simulink model "raspberrypi_robotaurus3"  (R2014a)
settings: Solver=FixedStepDiscrete  StartTime=0.0  StopTime=inf  RelTol=1e-3
undefined symbols (not defined in the file or in its folder): Rec, SDTV
libraries: embdlinuxlib x4, visionconversions x1
PreSaveFcn:
  | set_param(gcs, 'Location',[35 56 895 605])
settings Model: SimulationMode=external  ExtModeTrigDuration=100  Creator=The MathWorks Inc.  LastModifiedBy=Alejandro
settings DataIOCC: SignalLoggingSaveFormat=ModelDataLogs
settings OptimizationCC: ExpressionDepthLimit=2147483647  OptimizeModelRefInitCode=on  LifeSpan=Inf
settings DebuggingCC: UnderspecifiedInitializationDetection=Classic  SolverPrmCheckMsg=none  FcnCallInpInsideContextMsg=EnableAllAsWarning  StateNameClashWarn=warning
settings HardwareCC: ProdLargestAtomicInteger=Long  ProdLargestAtomicFloat=Double  ProdEndianess=LittleEndian  ProdHWDeviceType=ARM Compatible->ARM Cortex
settings RTWCC: SystemTargetFile=realtime.tlc  GenerateMakefile=off  TemplateMakefile=realtime.tmf  Description=Run on Target Hardware  RTWVerbose=off  ProcessScript=realtime_make_rtw_hook
settings CodeAppCC: CustomSymbolStrType=$N$R$M  InternalIdentifier=Classic
settings STFCustomTargetCC: TargetLibSuffix=.a  GenerateSampleERTMain=on  ConcurrentExecutionCompliant=off  GeneratePreprocessorConditionals=Use local settings  ERTCustomFileBanners=on  SupportNonInlinedSFcns=off  SupportVariableSizeSignals=on  MATLABClassNameForMDSCustomization=Simulink.SoftwareTarget.ERTCustomization  GRTInterface=off  SystemTargetFile=realtime.tlc
settings ERTTargetCC: CombineOutputUpdateFcns=off  SupportContinuousTime=on  SupportVariableSizeSignals=on  ExtMode=on  ExtModeMexArgs='169.254.0.2' 0 17725 5  ERTSrcFileBannerTemplate=realtime_code_template.cgt  ERTHdrFileBannerTemplate=realtime_code_template.cgt  ERTDataSrcFileTemplate=realtime_code_template.cgt  ERTDataHdrFileTemplate=realtime_code_template.cgt  ERTCustomFileTemplate=realtime_file_process.tlc

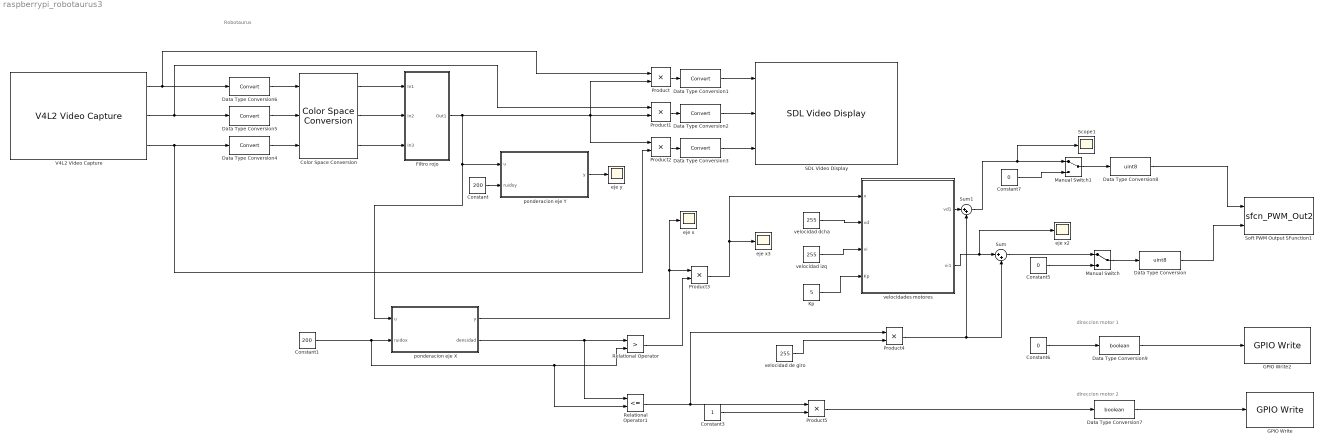
== system raspberrypi_robotaurus3 ==
  note: direccion motor 1
  note: direccion motor 2
  note: Robotaurus
  Color Space Conversion : visionconversions/Color Space  Conversion  conversion=Obsolete  conversionActive=R'G'B' to HSV  wp_str=D65  rec=Rec. 601 (SDTV)  sys=1125/60/2:1  imagePorts=Separate color signals
  Constant : Constant  Value=200
  Constant1 : Constant  Value=200
  Constant3 : Constant
  Constant5 : Constant  Value=0
  Constant6 : Constant  Value=0
  Constant7 : Constant  Value=0
  Data Type Conversion : DataTypeConversion  OutDataTypeStr=uint8
  Data Type Conversion{1..6} (6 alike) : DataTypeConversion
  Data Type Conversion7 : DataTypeConversion  OutDataTypeStr=boolean
  Data Type Conversion8 : DataTypeConversion  OutDataTypeStr=uint8
  Data Type Conversion9 : DataTypeConversion  OutDataTypeStr=boolean
  Filtro rojo : Subsystem
  GPIO Write : embdlinuxlib/GPIO Write  board=Model B Rev2  gpio=4  direction=Output  blockPlatform=Raspberry Pi
  GPIO Write2 : embdlinuxlib/GPIO Write  board=Model B Rev2  gpio=25  direction=Output  blockPlatform=Raspberry Pi
  Kp : Constant  Value=5
  Manual Switch : ManualSwitch
  Manual Switch1 : ManualSwitch
  Product{,1..5} (6 alike) : Product
  Relational Operator : RelationalOperator  Operator=>  OutDataTypeStr=boolean
  Relational Operator1 : RelationalOperator  Operator=<=  OutDataTypeStr=boolean
  SDL Video Display : embdlinuxlib/SDL Video Display  pixelFormat=RGB  pixelOrder=Planar  rowMajor=on  blockPlatform=Raspberry Pi
  Scope1 : Scope
      settings: YMin=200  YMax=255  SaveName=ScopeData3
  Soft PWM Output SFunction1 : S-Function  InitFcn=try, set_param(gcb,'FunctionName','sfcn_PWM_Out2'), end  FunctionName=sfcn_PWM_Out2  Parameters=uint8([0,12])  SFunctionModules=sfcn_PWM_Out2_wrapper  EnableBusSupport=off  mask(S-Function Builder){}
      mask init:
      | val = [[.9  0.75 0.75 1 1 .9 .9 1]',[1 1 0.75 0.75 .9 .9 1 .9]'];try , sys = get_param(gcb,'SfunBuilderFcnName');if isempty(sys), sys = get_param(gcb,'FunctionName'); end,catch, sys = get_param(gcb,'FunctionName'); end
      settings: CopyFcn=set_param(gcbh,'LinkStatus','none')  PreSaveFcn=try, set_param(gcb,'FunctionName','sfcn_PWM_Out2'), end  OpenFcn=sfunctionwizard(gcbh)
      mask Display: plot(val(:,1),val(:,2)),disp(sys), port_label('input',1,'motor1'), port_label('input',2,'motor2')
  Sum : Sum  Inputs=|++
  Sum1 : Sum  Inputs=|++
  V4L2 Video Capture : embdlinuxlib/V4L2 Video Capture  m_devName='/dev/video0'  roi=[0, 0, 640, 480]  imSizeSelection=160x120  imSize=[640, 480]  pixelFormat=RGB  pixelOrder=Planar  sampleTime=1/10  simOutput=Colorbars  blockPlatform=Raspberry Pi
  eje x : Scope
      settings: YMin=-50  YMax=35
  eje x2 : Scope
      settings: TimeRange=10  YMin=232.5  YMax=255  SaveName=ScopeData5
  eje x3 : Scope
      settings: YMin=-60  YMax=15  SaveName=ScopeData6
  eje y : Scope
      settings: YMin=-30  YMax=55
  ponderacion eje X : MATLAB Function  TreatAsAtomicUnit=on
  ponderacion eje Y : MATLAB Function  TreatAsAtomicUnit=on
  velocidad dcha : Constant  Value=255
  velocidad de giro : Constant  Value=255
  velocidad izq : Constant  Value=255
  velocidades motores : MATLAB Function  TreatAsAtomicUnit=on
  wires:
  V4L2 Video Capture/1 -> Product/1, Data Type Conversion6/1
  V4L2 Video Capture/2 -> Product1/1, Data Type Conversion5/1
  V4L2 Video Capture/3 -> Product2/2, Data Type Conversion4/1
  Color Space Conversion/1 -> Filtro rojo/1(In1)
  Color Space Conversion/2 -> Filtro rojo/2(In2)
  Color Space Conversion/3 -> Filtro rojo/3(In3)
  Data Type Conversion6/1 -> Color Space Conversion/1
  Filtro rojo/1(Out1) -> Product2/1, Product/2, Product1/2, ponderacion eje X/1(u), ponderacion eje Y/1(u)
  Data Type Conversion5/1 -> Color Space Conversion/2
  Data Type Conversion4/1 -> Color Space Conversion/3
  Product/1 -> Data Type Conversion1/1
  Product1/1 -> Data Type Conversion2/1
  Product2/1 -> Data Type Conversion3/1
  Data Type Conversion1/1 -> SDL Video Display/1
  Data Type Conversion2/1 -> SDL Video Display/2
  Data Type Conversion3/1 -> SDL Video Display/3
  ponderacion eje Y/1(y) -> eje y/1
  Constant/1 -> ponderacion eje Y/2(ruidoy)
  Constant1/1 -> Relational Operator1/2, Relational Operator/2, ponderacion eje X/2(ruidox)
  ponderacion eje X/2(densidad) -> Relational Operator1/1, Relational Operator/1
  ponderacion eje X/1(y) -> eje x/1, Product3/1
  velocidad izq/1 -> velocidades motores/3(vi)
  velocidad dcha/1 -> velocidades motores/2(vd)
  Constant3/1 -> Product5/2
  Data Type Conversion/1 -> Soft PWM Output SFunction1/2
  Constant5/1 -> Manual Switch/2
  Sum/1 -> Manual Switch/1
  Manual Switch/1 -> Data Type Conversion/1
  Data Type Conversion8/1 -> Soft PWM Output SFunction1/1
  Constant7/1 -> Manual Switch1/2
  Manual Switch1/1 -> Data Type Conversion8/1
  Relational Operator/1 -> Product3/2
  Relational Operator1/1 -> Product4/1, Product5/1
  velocidad de giro/1 -> Product4/2
  Data Type Conversion7/1 -> GPIO Write/1
  Product3/1 -> velocidades motores/1(x), eje x3/1
  Product4/1 -> Sum/2, Sum1/2
  velocidades motores/2(vi1) -> eje x2/1, Sum/1
  Data Type Conversion9/1 -> GPIO Write2/1
  Product5/1 -> Data Type Conversion7/1
  Constant6/1 -> Data Type Conversion9/1
  Sum1/1 -> Scope1/1, Manual Switch1/1
  velocidades motores/1(vd1) -> Sum1/1
  Kp/1 -> velocidades motores/4(Kp)

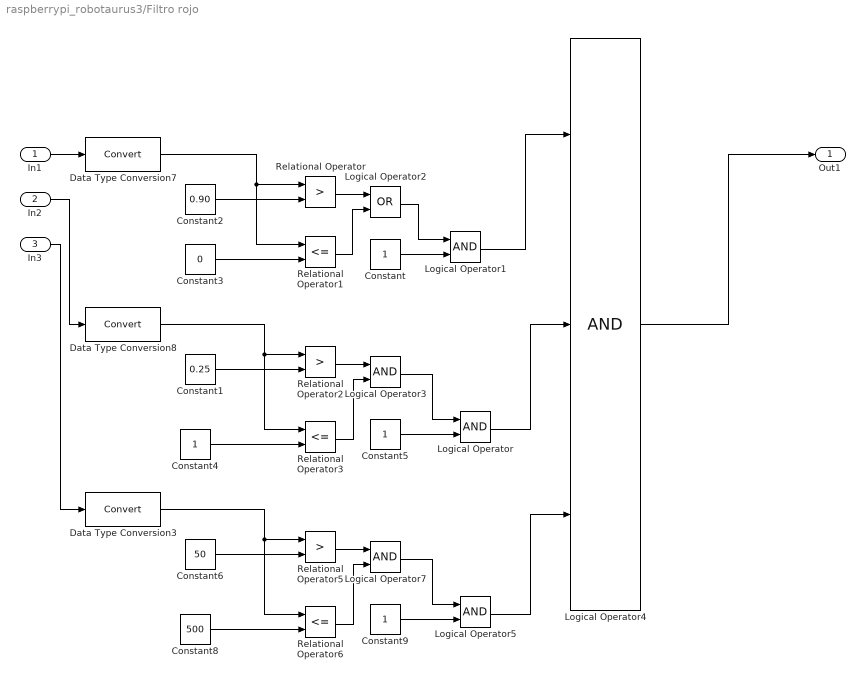
== system raspberrypi_robotaurus3/Filtro rojo ==
  In1 : Inport
  In2 : Inport  Port=2
  In3 : Inport  Port=3
  Constant{,4..5,9} (4 alike) : Constant
  Constant1 : Constant  Value=0.25
  Constant2 : Constant  Value=0.90
  Constant3 : Constant  Value=0
  Constant6 : Constant  Value=50
  Constant8 : Constant  Value=500
  Data Type Conversion3 : DataTypeConversion
  Data Type Conversion7 : DataTypeConversion
  Data Type Conversion8 : DataTypeConversion
  Logical Operator{,1,3,5,7} (5 alike) : Logic  AllPortsSameDT=off  OutDataTypeStr=boolean
  Logical Operator2 : Logic  Operator=OR  AllPortsSameDT=off  OutDataTypeStr=boolean
  Logical Operator4 : Logic  Inputs=3  AllPortsSameDT=off  OutDataTypeStr=boolean
  Relational Operator : RelationalOperator  Operator=>  OutDataTypeStr=boolean
  Relational Operator1 : RelationalOperator  Operator=<=  OutDataTypeStr=boolean
  Relational Operator2 : RelationalOperator  Operator=>  OutDataTypeStr=boolean
  Relational Operator3 : RelationalOperator  Operator=<=  OutDataTypeStr=boolean
  Relational Operator5 : RelationalOperator  Operator=>  OutDataTypeStr=boolean
  Relational Operator6 : RelationalOperator  Operator=<=  OutDataTypeStr=boolean
  Out1 : Outport
  wires:
  In1/1 -> Data Type Conversion7/1
  Relational Operator/1 -> Logical Operator2/1
  Relational Operator1/1 -> Logical Operator2/2
  Constant2/1 -> Relational Operator/2
  Constant3/1 -> Relational Operator1/2
  In2/1 -> Data Type Conversion8/1
  Logical Operator1/1 -> Logical Operator4/1
  Constant/1 -> Logical Operator1/2
  Data Type Conversion7/1 -> Relational Operator1/1, Relational Operator/1
  Logical Operator2/1 -> Logical Operator1/1
  Relational Operator2/1 -> Logical Operator3/1
  Relational Operator3/1 -> Logical Operator3/2
  Data Type Conversion8/1 -> Relational Operator3/1, Relational Operator2/1
  Logical Operator3/1 -> Logical Operator/1
  Constant5/1 -> Logical Operator/2
  Constant1/1 -> Relational Operator2/2
  Constant4/1 -> Relational Operator3/2
  Logical Operator/1 -> Logical Operator4/2
  Relational Operator5/1 -> Logical Operator7/1
  Relational Operator6/1 -> Logical Operator7/2
  Data Type Conversion3/1 -> Relational Operator6/1, Relational Operator5/1
  Logical Operator7/1 -> Logical Operator5/1
  Constant9/1 -> Logical Operator5/2
  Constant6/1 -> Relational Operator5/2
  Constant8/1 -> Relational Operator6/2
  Logical Operator5/1 -> Logical Operator4/3
  In3/1 -> Data Type Conversion3/1
  Logical Operator4/1 -> Out1/1

== matlab function raspberrypi_robotaurus3/ponderacion eje X ==
  data: u input; y output; ruidox input; densidad output
function [y,densidad] = horizontal(u, ruidox)
%#codegen
f=sum(u');
barrimola=sum(f); %suma de unos
if (barrimola<=ruidox) barrimola = 0;
end
v=1:1:(size(f,2)/2);
w=(-size(f,2)/2):1:-1;
x=[w v]; %eje x
zenermola=f.*x; %vector de las medias
y = sum(zenermola)/barrimola; 
densidad= barrimola;

== matlab function raspberrypi_robotaurus3/ponderacion eje Y ==
  data: u input; y output; ruidoy input
function y = horizontal(u, ruidoy)
%#codegen
f=sum(u);
barrimola=sum(f); %suma de unos
if (barrimola<=ruidoy) barrimola = 0;
end
v=1:1:(size(f,2)/2);
w=(-size(f,2)/2):1:-1;
x=[w v]; %eje x
zenermola=f.*x; %vector de las medias
y = sum(zenermola)/barrimola;

== matlab function raspberrypi_robotaurus3/velocidades motores ==
  data: vd1 output; x input; vd input; vi input; vi1 output; Kp input
function [vd1, vi1] = velocidades(x, vd, vi, Kp)
%#codegen
coordenada = x;
velocidad_derecha =0;
velocidad_izquierda = 0;
   if(coordenada==0)
    velocidad_derecha=vd;
    velocidad_izquierda=vi;
   else
   end
   if(coordenada<0)
   velocidad_izquierda=(coordenada*Kp+vd);
    velocidad_derecha=vd;  %si el punto se desplaza a la izq, vi más lento
   else
   end
   if(coordenada>0)
    velocidad_izquierda=vi;
    velocidad_derecha=(vi-coordenada*Kp);
   else
   end 
  vd1= velocidad_derecha;
  vi1 = velocidad_izquierda;
end
